simulink model "eCS_Algo_Simulation_2015b_opti - Copy"  (R2015b)
settings: Solver=ode1  StartTime=0.0  StopTime=3  FixedStep=1/80000  RelTol=1e-3
PreLoadFcn:
  | if exist('tl_preloadfcn','file'), tl_preloadfcn(gcs,402); end
PostLoadFcn:
  | , if any(exist('dsrtsu_mdlpostloadfcn', 'file') == [2, 3, 6]), try dsrtsu_mdlpostloadfcn('Execute', bdroot); catch fprintf('Error in PostLoadFcn (dsrtsu_mdlpostloadfcn) for model "%s":\n %s\n', bdroot, lasterr); end, end,
  | if exist('tl_postloadfcn','file'), tl_postloadfcn(gcs,402); end
InitFcn:
  | Omegan=1.3024e+03;
  | xi=0.9; %0.48
  | K=0.1931;
  | K1=0.0198;
  | TauLocked=0.00255;
  | TauUnLocked=0.0042;
  | Kp=1/(2*K1);
  | Ki=Kp/((TauLocked+TauUnLocked)/2);
  | if exist('tlds_init','file'), tlds_init(gcs); end
StartFcn:
  | if exist('tlds_start','file'), tlds_start(gcs); end
StopFcn:
  | if exist('tlds_stop','file'), tlds_stop(gcs); end
model workspace (MAT data in the model file):
  au8PrevExecProfile = [0 0 0 0 0 0]
values from neighbouring files (symbols this model uses):
  AccSensor = 5    [Parameter_eCS_Algo.m]
  AlgoType = 0    [Parameter_eCS_Algo.m]
  Cxy = 1*0.017    (= 0.017)    [Acc_Init_SelV1.m]
  Cxz = 1*0.017    (= 0.017)    [Acc_Init_SelV1.m]
  Cyx = 1*0.017    (= 0.017)    [Acc_Init_SelV1.m]
  Cyz = 1*0.017    (= 0.017)    [Acc_Init_SelV1.m]
  Czx = 1*0.017    (= 0.017)    [Acc_Init_SelV1.m]
  Czy = 1*0.017    (= 0.017)    [Acc_Init_SelV1.m]
  Forced_Oscillation = 0    [Parameter_eCS_Algo.m]    (also in run_Rotation_sim.m = run)
  FreqTemperature = 10    [Acc_Init_SelV1.m]
  MaxSensorOffset = 0.3    [Acc_Init_SelV1.m]
  Mean_x_noise = 4e-3    (= 0.004)    [Acc_Init_SelV1.m]
  Mean_y_noise = 4e-3    (= 0.004)    [Acc_Init_SelV1.m]
  Mean_z_noise = 4e-3    (= 0.004)    [Acc_Init_SelV1.m]
  ODR = 8000    [Acc_Init_SelV1.m]
  offsetcorrection_on_off = 0    [Parameter_eCS_Algo.m]
  phi_pulse_rotation = 0    [Parameter_eCS_Algo.m]    (also in run_Rotation_sim.m = angle)
  pulsetype = 2    [Parameter_eCS_Algo.m]    (also in run_simulation.m = j; run_simulation_ActiveX.m = j)
  Range = 4    [Acc_Init_SelV1.m]
  sensitivity_optimisation = 0    [Parameter_eCS_Algo.m]
  TempBias = 0    [Acc_Init_SelV1.m]
  TemperatureAmp = 0    [Acc_Init_SelV1.m]
  Var_x_noise = 1.84e-9    (= 1.84e-09)    [Acc_Init_SelV1.m]
  Var_y_noise = 2.025e-09    [Acc_Init_SelV1.m]
  Var_z_noise = 1.374e-09    [Acc_Init_SelV1.m]
  w_x = 2*pi*F_x    (= 376.991118431)    [Acc_Init_SelV1.m]
  w_y = 2*pi*F_y    (= 376.991118431)    [Acc_Init_SelV1.m]
  w_z = 2*pi*F_z    (= 376.991118431)    [Acc_Init_SelV1.m]
  x_max_temp_drift = 0.061    [Acc_Init_SelV1.m]
  x_offset_enable = 0    [Acc_Init_SelV1.m]
  x_run_to_run_drift = 0.0    (= 0)    [Acc_Init_SelV1.m]
  x_temp_co_drift = 0.000    (= 0)    [Acc_Init_SelV1.m]
  Xi_x = 0.7    [Acc_Init_SelV1.m]
  Xi_y = 0.7    [Acc_Init_SelV1.m]
  Xi_z = 0.7    [Acc_Init_SelV1.m]
  y_max_temp_drift = 0.061    [Acc_Init_SelV1.m]
  y_offset_enable = 0    [Acc_Init_SelV1.m]
  y_run_to_run_drift = 0.0    (= 0)    [Acc_Init_SelV1.m]
  y_temp_co_drift = 0.000    (= 0)    [Acc_Init_SelV1.m]
  z_max_temp_drift = 0.13    [Acc_Init_SelV1.m]
  z_offset_enable = 0    [Acc_Init_SelV1.m]
  z_run_to_run_drift = 0.0    (= 0)    [Acc_Init_SelV1.m]
  z_temp_co_drift = 0.000    (= 0)    [Acc_Init_SelV1.m]
undefined symbols (not defined in the file or in its folder): ddv, DiscIntNeverNeededParam, gmw_roada_x__m_s__, gmw_roada_y__m_s__, gmw_roadtime_2kHz, KSF_50_a_x, KSF_50_a_y, KSF_50_time, KSG_30_a_x, KSG_30_a_y, KSG_30_time, Meldorf_HindenburgstraAcceleration_x__m_s_2_, Meldorf_HindenburgstraAcceleration_y__m_s_2_, Meldorf_HindenburgstraAcceleration_z__m_s_2_, Meldorf_HindenburgstraTime__s_, pulse_FF27, pulse_MPDB, pulse_ODB40, pulse_ODB64, pulse_USNCAP, pulsetime_FF27, pulsetime_MPDB, pulsetime_ODB40, pulsetime_ODB64, pulsetime_USNCAP, Rauasphalt_60_a_x, Rauasphalt_60_a_y, Rauasphalt_60_time, sigbuilder_block, VW_416_2kHza_x_2kHz, VW_416_2kHza_y_2kHz, VW_416_2kHztime_2kHz
libraries: tllib x22, simulink x20, tl_autosar_lib x10, simulink_extras x7, LIB_TF_G_12_StepControl x2, LIB_TF_G_111 x1, LIB_TF_G_112 x1
(part 3 of 9)

== system eCS_Algo_Simulation_2015b_opti - Copy/FSM/Subsystem/FSM/FSM/FSM_runMainFunction ==
  drparg_b8EcsFlag : Inport  PortDimensions=1  mask(TL_Inport){data={'autosar',{'useautosarcommunication',1,'senderreceiverport','prrEcsAlgoFlag','dataelement','b8EcsFlag'},'date',738304.65103487263}}
      settings: CopyFcn=if exist('tl_reset_reviewflag') == 2, tl_reset_reviewflag(gcbh); end  DeleteFcn=if exist('delete_tlblock','file')==2,delete_tlblock(gcbh);end  NameChangeFcn=if exist('rename_tlblock','file')==2,rename_tlblock(gcbh);end  OpenFcn=if exist('tl_open_blockdlg','file')==2,tl_open_blockdlg(gcbh);else,open_system(gcbh,'parameter');end
      mask Help: eval(['if exist(''tl_online_help'',''file'') == 2, tl_online_help(''Topic'',''TL_Inport''),else, web([''jar:file:///'',matlabroot,''/help/toolbox/simulink/help.jar!/slref/' lower(get_param(gcbh,'Blocktype')) '.html''], ''-helpbrowser''),end'])
      mask Display: plot([0.2 0.35 NaN 0.65 0.8],[0 1 NaN 0 1]);
  bModeStatus : Inport  Port=2  PortDimensions=1  mask(TL_Inport){data={'autosar',{'useautosarcommunication',1,'kind',3,'interrunnablevariable','FSM_b8_ModeStatusResult','serverport','pseModeManagement'},'date',738785.60019108793}}
      settings: CopyFcn=if exist('tl_reset_reviewflag','file')==2,tl_reset_reviewflag(gcbh);end  DeleteFcn=if exist('delete_tlblock','file')==2,delete_tlblock(gcbh);end  NameChangeFcn=if exist('rename_tlblock','file')==2,rename_tlblock(gcbh);end  OpenFcn=if exist('tl_open_blockdlg','file')==2,tl_open_blockdlg(gcbh);else,open_system(gcbh,'parameter');end
      mask Help: eval(['if exist(''tl_online_help'',''file'') == 2, tl_online_help(''Topic'',''TL_Inport''),else, web([''jar:file:///'',matlabroot,''/help/toolbox/simulink/help.jar!/slref/' lower(get_param(gcbh,'Blocktype')) '.html''], ''-helpbrowser''),end'])
      mask Display: plot([0.2 0.35 NaN 0.65 0.8],[0 1 NaN 0 1]);
  ab8IsSolenoidUsed : Inport  Port=3  PortDimensions=6  mask(TL_Inport){data={'autosar',{'useautosarcommunication',1,'kind',3,'interrunnablevariable','ab8IsSolenoidUsed'},'date',738307.71878736117}}
      settings: CopyFcn=if exist('tl_reset_reviewflag') == 2, tl_reset_reviewflag(gcbh); end  DeleteFcn=if exist('delete_tlblock','file')==2,delete_tlblock(gcbh);end  NameChangeFcn=if exist('rename_tlblock','file')==2,rename_tlblock(gcbh);end  OpenFcn=if exist('tl_open_blockdlg','file')==2,tl_open_blockdlg(gcbh);else,open_system(gcbh,'parameter');end
      mask Help: eval(['if exist(''tl_online_help'',''file'') == 2, tl_online_help(''Topic'',''TL_Inport''),else, web([''jar:file:///'',matlabroot,''/help/toolbox/simulink/help.jar!/slref/' lower(get_param(gcbh,'Blocktype')) '.html''], ''-helpbrowser''),end'])
      mask Display: plot([0.2 0.35 NaN 0.65 0.8],[0 1 NaN 0 1]);
  Constant2 : Constant  Commented=on  Value=2  mask(TL_Constant){data={'date',738673.71713201387}}
      settings: CopyFcn=if exist('tl_reset_reviewflag') == 2, tl_reset_reviewflag(gcbh); end  DeleteFcn=if exist('delete_tlblock','file')==2,delete_tlblock(gcbh);end  NameChangeFcn=if exist('rename_tlblock','file')==2,rename_tlblock(gcbh);end  OpenFcn=if exist('tl_open_blockdlg','file')==2,tl_open_blockdlg(gcbh);else,open_system(gcbh,'parameter');end
      mask Help: eval(['if exist(''tl_online_help'',''file'') == 2, tl_online_help(''Topic'',''TL_Constant''),else, web([''jar:file:///'',matlabroot,''/help/toolbox/simulink/help.jar!/slref/' lower(get_param(gcbh,'Blocktype')) '.html''], ''-helpbrowser''),end'])
      mask Display: plot([-0.1, 1.05, NaN, -0.1, 1.05],[.01, .01, NaN, .99, .99]);
  Constant3 : Constant  Commented=on  Value=10  mask(TL_Constant){data={'date',738673.718190243}}
      settings: CopyFcn=if exist('tl_reset_reviewflag') == 2, tl_reset_reviewflag(gcbh); end  DeleteFcn=if exist('delete_tlblock','file')==2,delete_tlblock(gcbh);end  NameChangeFcn=if exist('rename_tlblock','file')==2,rename_tlblock(gcbh);end  OpenFcn=if exist('tl_open_blockdlg','file')==2,tl_open_blockdlg(gcbh);else,open_system(gcbh,'parameter');end
      mask Help: eval(['if exist(''tl_online_help'',''file'') == 2, tl_online_help(''Topic'',''TL_Constant''),else, web([''jar:file:///'',matlabroot,''/help/toolbox/simulink/help.jar!/slref/' lower(get_param(gcbh,'Blocktype')) '.html''], ''-helpbrowser''),end'])
      mask Display: plot([-0.1, 1.05, NaN, -0.1, 1.05],[.01, .01, NaN, .99, .99]);
  Determine Transition : Subsystem  TreatAsAtomicUnit=on
  ExecuteState : Subsystem  TreatAsAtomicUnit=on
  Logical Operator : Logic  Commented=on  Operator=OR  AllPortsSameDT=off  OutDataTypeStr=boolean  mask(TL_LogicalOperator){data={'date',738673.70713811344}}
      settings: DeleteFcn=if exist('delete_tlblock','file')==2,delete_tlblock(gcbh);end  NameChangeFcn=if exist('rename_tlblock','file')==2,rename_tlblock(gcbh);end  OpenFcn=if exist('tl_open_blockdlg','file')==2,tl_open_blockdlg(gcbh);else,open_system(gcbh,'parameter');end
      mask Help: eval(['if exist(''tl_online_help'',''file'') == 2, tl_online_help(''Topic'',''TL_LogicalOperator''),else, web([''jar:file:///'',matlabroot,''/help/toolbox/simulink/help.jar!/slref/' lower(get_param(gcbh,'Blocktype')) '.html''], ''-helpbrowser''),end'])
      mask Display: plot([-0.1, 1.05, NaN, -0.1, 1.05],[.01, .01, NaN, .99, .99]);
  Relational Operator : RelationalOperator  Commented=on  Operator===  OutDataTypeStr=boolean  mask(TL_RelationalOperator){data={'date',738673.58053900464}}
      settings: DeleteFcn=if exist('delete_tlblock','file')==2,delete_tlblock(gcbh);end  NameChangeFcn=if exist('rename_tlblock','file')==2,rename_tlblock(gcbh);end  OpenFcn=if exist('tl_open_blockdlg','file')==2,tl_open_blockdlg(gcbh);else,open_system(gcbh,'parameter');end
      mask Help: eval(['if exist(''tl_online_help'',''file'') == 2, tl_online_help(''Topic'',''TL_RelationalOperator''),else, web([''jar:file:///'',matlabroot,''/help/toolbox/simulink/help.jar!/slref/' lower(get_param(gcbh,'Blocktype')) '.html''], ''-helpbrowser''),end'])
      mask Display: plot([-0.1, 1.05, NaN, -0.1, 1.05],[.01, .01, NaN, .99, .99]);
  Relational Operator1 : RelationalOperator  Commented=on  Operator===  OutDataTypeStr=boolean  mask(TL_RelationalOperator){data={'date',738673.58053900464}}
      settings: DeleteFcn=if exist('delete_tlblock','file')==2,delete_tlblock(gcbh);end  NameChangeFcn=if exist('rename_tlblock','file')==2,rename_tlblock(gcbh);end  OpenFcn=if exist('tl_open_blockdlg','file')==2,tl_open_blockdlg(gcbh);else,open_system(gcbh,'parameter');end
      mask Help: eval(['if exist(''tl_online_help'',''file'') == 2, tl_online_help(''Topic'',''TL_RelationalOperator''),else, web([''jar:file:///'',matlabroot,''/help/toolbox/simulink/help.jar!/slref/' lower(get_param(gcbh,'Blocktype')) '.html''], ''-helpbrowser''),end'])
      mask Display: plot([-0.1, 1.05, NaN, -0.1, 1.05],[.01, .01, NaN, .99, .99]);
  Runnable : tllib/Function  data={'autosar',{'useautosarspecification',1,'softwarecomponent','AUTOLIV/SoftwareComponents/FSM/FSM','runnable','FSM_runMainFunction'},'date',738304.65103259264}  displayString=RUNNABLE
  Src2 : Subsystem  Commented=on
  old state : UnitDelay  InitialCondition=ddv('FSM/astFsm/Components/au8FsmStatesOld')  SampleTime=-1  mask(TL_UnitDelay){data={'output',{'name','$D','inheritscaling',1},'state',{'variable','FSM/astFsm/Components/au8FsmStatesOld'},'date',738331.66886591434}}
      settings: CopyFcn=if exist('tl_reset_reviewflag') == 2, tl_reset_reviewflag(gcbh); end  DeleteFcn=if exist('delete_tlblock','file')==2,delete_tlblock(gcbh);end  NameChangeFcn=if exist('rename_tlblock','file')==2,rename_tlblock(gcbh);end  OpenFcn=if exist('tl_open_blockdlg','file')==2,tl_open_blockdlg(gcbh);else,open_system(gcbh,'parameter');end
      mask Help: eval(['if exist(''tl_online_help'',''file'') == 2, tl_online_help(''Topic'',''TL_UnitDelay''),else, web([''jar:file:///'',matlabroot,''/help/toolbox/simulink/help.jar!/slref/' lower(get_param(gcbh,'Blocktype')) '.html''], ''-helpbrowser''),end'])
      mask Display: plot([-0.1, 1.05, NaN, -0.1, 1.05],[.01, .01, NaN, .99, .99]);
  scp_KL30_OV_GetTestResult : Subsystem  Commented=on  TreatAsAtomicUnit=on
  scp_KL30_UV_GetTestResult : Subsystem  Commented=on  TreatAsAtomicUnit=on
  au8FsmState : Outport  PortDimensions=6  mask(TL_Outport){data={'logdata',{'loggingmode',1},'autosar',{'useautosarcommunication',1,'senderreceiverport','psrSolenoidState','dataelement','au8SolenoidState'},'date',738314.63122943288}}
      settings: CopyFcn=if exist('tl_reset_reviewflag') == 2, tl_reset_reviewflag(gcbh); end  DeleteFcn=if exist('delete_tlblock','file')==2,delete_tlblock(gcbh);end  NameChangeFcn=if exist('rename_tlblock','file')==2,rename_tlblock(gcbh);end  OpenFcn=if exist('tl_open_blockdlg','file')==2,tl_open_blockdlg(gcbh);else,open_system(gcbh,'parameter');end
      mask Help: eval(['if exist(''tl_online_help'',''file'') == 2, tl_online_help(''Topic'',''TL_Outport''),else, web([''jar:file:///'',matlabroot,''/help/toolbox/simulink/help.jar!/slref/' lower(get_param(gcbh,'Blocktype')) '.html''], ''-helpbrowser''),end'])
      mask Display: plot([0.2 0.35 NaN 0.65 0.8],[0 1 NaN 0 1]);
  au8SelectedProfile : Outport  Port=2  PortDimensions=6  mask(TL_Outport){data={'logdata',{'loggingmode',1},'autosar',{'useautosarcommunication',1,'senderreceiverport','psrSolenoidProfile','dataelement','au8SelectedProfile'},'date',738785.47525618051}}
      settings: CopyFcn=if exist('tl_reset_reviewflag') == 2, tl_reset_reviewflag(gcbh); end  DeleteFcn=if exist('delete_tlblock','file')==2,delete_tlblock(gcbh);end  NameChangeFcn=if exist('rename_tlblock','file')==2,rename_tlblock(gcbh);end  OpenFcn=if exist('tl_open_blockdlg','file')==2,tl_open_blockdlg(gcbh);else,open_system(gcbh,'parameter');end
      mask Help: eval(['if exist(''tl_online_help'',''file'') == 2, tl_online_help(''Topic'',''TL_Outport''),else, web([''jar:file:///'',matlabroot,''/help/toolbox/simulink/help.jar!/slref/' lower(get_param(gcbh,'Blocktype')) '.html''], ''-helpbrowser''),end'])
      mask Display: plot([0.2 0.35 NaN 0.65 0.8],[0 1 NaN 0 1]);
  wires:
  drparg_b8EcsFlag/1 -> Determine Transition/1(b8EcsFlag)
  ab8IsSolenoidUsed/1 -> Determine Transition/2(ab8IsSolenoidUsed)
  Determine Transition/1(au8State) -> old state/1, ExecuteState/1(au8States), au8FsmState/1
  ExecuteState/1(au8FsmProfiles) -> au8SelectedProfile/1
  old state/1 -> Determine Transition/3(au8OldState)
  Src2/1(u8AutoTestId) -> scp_KL30_OV_GetTestResult/1(u8AutoTestId)
  scp_KL30_OV_GetTestResult/1(u8TestResult) -> Relational Operator/1
  Constant2/1 -> Relational Operator1/1, Relational Operator/2
  scp_KL30_UV_GetTestResult/1(u8TestResult) -> Relational Operator1/2
  Constant3/1 -> scp_KL30_UV_GetTestResult/1(u8AutoTestId)
  Relational Operator/1 -> Logical Operator/1
  Relational Operator1/1 -> Logical Operator/2
  bModeStatus/1 -> Determine Transition/4(bModeStatus)

== system eCS_Algo_Simulation_2015b_opti - Copy/SAD/Subsystem/SAD/SAD/SAD_Init ==
  BusCreator : BusCreator  Inputs=2
  BusCreator1 : BusCreator  Inputs=2
  Constant : Constant  Value=ddv('DIOIF/Macros/IO_Level/DIOIF_STD_HIGH')  mask(TL_Constant){data={'output',{'variable','DIOIF/Macros/IO_Level/DIOIF_STD_HIGH'},'date',738597.36695635412}}
      settings: CopyFcn=if exist('tl_reset_reviewflag') == 2, tl_reset_reviewflag(gcbh); end  DeleteFcn=if exist('delete_tlblock','file')==2,delete_tlblock(gcbh);end  NameChangeFcn=if exist('rename_tlblock','file')==2,rename_tlblock(gcbh);end  OpenFcn=if exist('tl_open_blockdlg','file')==2,tl_open_blockdlg(gcbh);else,open_system(gcbh,'parameter');end
      mask Help: eval(['if exist(''tl_online_help'',''file'') == 2, tl_online_help(''Topic'',''TL_Constant''),else, web([''jar:file:///'',matlabroot,''/help/toolbox/simulink/help.jar!/slref/' lower(get_param(gcbh,'Blocktype')) '.html''], ''-helpbrowser''),end'])
      mask Display: plot([-0.1, 1.05, NaN, -0.1, 1.05],[.01, .01, NaN, .99, .99]);
  Constant1 : Constant  Value=ddv('DIOIF/Macros/Channels/DIOIF_CH_EN_BOOST')  mask(TL_Constant){data={'output',{'variable','DIOIF/Macros/Channels/DIOIF_CH_EN_BOOST'},'date',738597.36719569447}}
      settings: CopyFcn=if exist('tl_reset_reviewflag') == 2, tl_reset_reviewflag(gcbh); end  DeleteFcn=if exist('delete_tlblock','file')==2,delete_tlblock(gcbh);end  NameChangeFcn=if exist('rename_tlblock','file')==2,rename_tlblock(gcbh);end  OpenFcn=if exist('tl_open_blockdlg','file')==2,tl_open_blockdlg(gcbh);else,open_system(gcbh,'parameter');end
      mask Help: eval(['if exist(''tl_online_help'',''file'') == 2, tl_online_help(''Topic'',''TL_Constant''),else, web([''jar:file:///'',matlabroot,''/help/toolbox/simulink/help.jar!/slref/' lower(get_param(gcbh,'Blocktype')) '.html''], ''-helpbrowser''),end'])
      mask Display: plot([-0.1, 1.05, NaN, -0.1, 1.05],[.01, .01, NaN, .99, .99]);
  Constant2 : Constant  Value=ddv('DIOIF/Macros/IO_Level/DIOIF_STD_HIGH')  mask(TL_Constant){data={'output',{'variable','DIOIF/Macros/IO_Level/DIOIF_STD_HIGH'},'date',738597.36695635412}}
      settings: CopyFcn=if exist('tl_reset_reviewflag') == 2, tl_reset_reviewflag(gcbh); end  DeleteFcn=if exist('delete_tlblock','file')==2,delete_tlblock(gcbh);end  NameChangeFcn=if exist('rename_tlblock','file')==2,rename_tlblock(gcbh);end  OpenFcn=if exist('tl_open_blockdlg','file')==2,tl_open_blockdlg(gcbh);else,open_system(gcbh,'parameter');end
      mask Help: eval(['if exist(''tl_online_help'',''file'') == 2, tl_online_help(''Topic'',''TL_Constant''),else, web([''jar:file:///'',matlabroot,''/help/toolbox/simulink/help.jar!/slref/' lower(get_param(gcbh,'Blocktype')) '.html''], ''-helpbrowser''),end'])
      mask Display: plot([-0.1, 1.05, NaN, -0.1, 1.05],[.01, .01, NaN, .99, .99]);
  Constant3 : Constant  Value=ddv('DIOIF/Macros/Channels/DIOIF_CH_EN_BOOST_2')  mask(TL_Constant){data={'output',{'variable','DIOIF/Macros/Channels/DIOIF_CH_EN_BOOST_2'},'date',738597.36739057873}}
      settings: CopyFcn=if exist('tl_reset_reviewflag') == 2, tl_reset_reviewflag(gcbh); end  DeleteFcn=if exist('delete_tlblock','file')==2,delete_tlblock(gcbh);end  NameChangeFcn=if exist('rename_tlblock','file')==2,rename_tlblock(gcbh);end  OpenFcn=if exist('tl_open_blockdlg','file')==2,tl_open_blockdlg(gcbh);else,open_system(gcbh,'parameter');end
      mask Help: eval(['if exist(''tl_online_help'',''file'') == 2, tl_online_help(''Topic'',''TL_Constant''),else, web([''jar:file:///'',matlabroot,''/help/toolbox/simulink/help.jar!/slref/' lower(get_param(gcbh,'Blocktype')) '.html''], ''-helpbrowser''),end'])
      mask Display: plot([-0.1, 1.05, NaN, -0.1, 1.05],[.01, .01, NaN, .99, .99]);
  Runnable : tllib/Function  data={'autosar',{'useautosarspecification',1,'softwarecomponent','AUTOLIV/SoftwareComponents/SAD/SAD','runnable','SAD_Init'},'date',738422.45749591431}  displayString=RUNNABLE
  EN_Boost_1 : Outport  mask(TL_BusOutport){data={'#autoscaling',2,'#message',2,'#output',2,'#logdata',2,'signals',{{'WriteChannel',{'u8ChannelID';'u8Level'}}},'autosar',{'useautosarcommunication',1,'kind',4,'clientserverport','pclDioIfServices','operation','WriteChannel'},'date',738430.41690740746}}
      settings: CopyFcn=if exist('tl_reset_reviewflag') == 2, tl_reset_reviewflag(gcbh); end  DeleteFcn=if exist('delete_tlblock','file')==2,delete_tlblock(gcbh);end  NameChangeFcn=if exist('rename_tlblock','file')==2,rename_tlblock(gcbh);end  OpenFcn=if exist('tl_open_blockdlg','file')==2,tl_open_blockdlg(gcbh);else,open_system(gcbh,'parameter');end
      mask Help: eval(['if exist(''tl_online_help'',''file'') == 2, tl_online_help(''Topic'',''TL_Outport''),else, web([''jar:file:///'',matlabroot,''/help/toolbox/simulink/help.jar!/slref/' lower(get_param(gcbh,'Blocktype')) '.html''], ''-helpbrowser''),end'])
      mask Display: plot([0.2 0.35 NaN 0.65 0.8],[0 1 NaN 0 1]);
  EN_Boost_2 : Outport  Port=2  mask(TL_BusOutport){data={'#autoscaling',2,'#message',2,'#output',2,'#logdata',2,'signals',{{'WriteChannel',{'u8ChannelID';'u8Level'}}},'autosar',{'useautosarcommunication',1,'kind',4,'clientserverport','pclDioIfServices','operation','WriteChannel'},'date',738430.41690740746}}
      settings: CopyFcn=if exist('tl_reset_reviewflag') == 2, tl_reset_reviewflag(gcbh); end  DeleteFcn=if exist('delete_tlblock','file')==2,delete_tlblock(gcbh);end  NameChangeFcn=if exist('rename_tlblock','file')==2,rename_tlblock(gcbh);end  OpenFcn=if exist('tl_open_blockdlg','file')==2,tl_open_blockdlg(gcbh);else,open_system(gcbh,'parameter');end
      mask Help: eval(['if exist(''tl_online_help'',''file'') == 2, tl_online_help(''Topic'',''TL_Outport''),else, web([''jar:file:///'',matlabroot,''/help/toolbox/simulink/help.jar!/slref/' lower(get_param(gcbh,'Blocktype')) '.html''], ''-helpbrowser''),end'])
      mask Display: plot([0.2 0.35 NaN 0.65 0.8],[0 1 NaN 0 1]);
  wires:
  Constant1/1 -> BusCreator/1  "u8ChannelID"
  Constant/1 -> BusCreator/2  "u8Level"
  BusCreator/1 -> EN_Boost_1/1  "WriteChannel"
  Constant3/1 -> BusCreator1/1  "u8ChannelID"
  Constant2/1 -> BusCreator1/2  "u8Level"
  BusCreator1/1 -> EN_Boost_2/1  "WriteChannel"

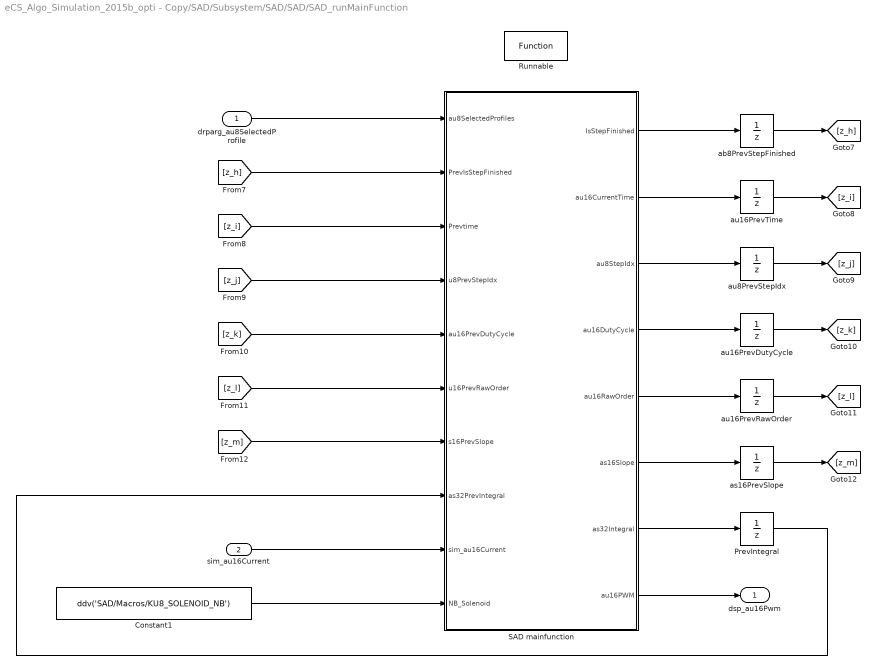
== system eCS_Algo_Simulation_2015b_opti - Copy/SAD/Subsystem/SAD/SAD/SAD_runMainFunction ==
  drparg_au8SelectedProfile : Inport  PortDimensions=6  mask(TL_Inport){data={'logdata',{'loggingmode',1},'autosar',{'useautosarcommunication',1,'senderreceiverport','prrFsmProfile','dataelement','au8SelectedProfile'},'date',738567.35573128471}}
      settings: CopyFcn=if exist('tl_reset_reviewflag') == 2, tl_reset_reviewflag(gcbh); end  DeleteFcn=if exist('delete_tlblock','file')==2,delete_tlblock(gcbh);end  NameChangeFcn=if exist('rename_tlblock','file')==2,rename_tlblock(gcbh);end  OpenFcn=if exist('tl_open_blockdlg','file')==2,tl_open_blockdlg(gcbh);else,open_system(gcbh,'parameter');end
      mask Help: eval(['if exist(''tl_online_help'',''file'') == 2, tl_online_help(''Topic'',''TL_Inport''),else, web([''jar:file:///'',matlabroot,''/help/toolbox/simulink/help.jar!/slref/' lower(get_param(gcbh,'Blocktype')) '.html''], ''-helpbrowser''),end'])
      mask Display: plot([0.2 0.35 NaN 0.65 0.8],[0 1 NaN 0 1]);
  sim_au16Current : Inport  Port=2
  Constant1 : Constant  Value=ddv('SAD/Macros/KU8_SOLENOID_NB')  mask(TL_Constant){data={'output',{'variable','SAD/Macros/KU8_SOLENOID_NB'},'date',738430.41690414352}}
      settings: CopyFcn=if exist('tl_reset_reviewflag') == 2, tl_reset_reviewflag(gcbh); end  DeleteFcn=if exist('delete_tlblock','file')==2,delete_tlblock(gcbh);end  NameChangeFcn=if exist('rename_tlblock','file')==2,rename_tlblock(gcbh);end  OpenFcn=if exist('tl_open_blockdlg','file')==2,tl_open_blockdlg(gcbh);else,open_system(gcbh,'parameter');end
      mask Help: eval(['if exist(''tl_online_help'',''file'') == 2, tl_online_help(''Topic'',''TL_Constant''),else, web([''jar:file:///'',matlabroot,''/help/toolbox/simulink/help.jar!/slref/' lower(get_param(gcbh,'Blocktype')) '.html''], ''-helpbrowser''),end'])
      mask Display: plot([-0.1, 1.05, NaN, -0.1, 1.05],[.01, .01, NaN, .99, .99]);
  PrevIntegral : UnitDelay  InitialCondition=ddv('SAD/Vars/Steps/as32PrevIntegral')  SampleTime=-1  mask(TL_UnitDelay){data={'output',{'description',['Resolution:  2^-15'],'name','$D','type','Int32','scaling','scPID'},'state',{'variable','SAD/Vars/Steps/as32PrevIntegral'},'date',738672.58140456013}}
      settings: CopyFcn=if exist('tl_reset_reviewflag') == 2, tl_reset_reviewflag(gcbh); end  DeleteFcn=if exist('delete_tlblock','file')==2,delete_tlblock(gcbh);end  NameChangeFcn=if exist('rename_tlblock','file')==2,rename_tlblock(gcbh);end  OpenFcn=if exist('tl_open_blockdlg','file')==2,tl_open_blockdlg(gcbh);else,open_system(gcbh,'parameter');end
      mask Help: eval(['if exist(''tl_online_help'',''file'') == 2, tl_online_help(''Topic'',''TL_UnitDelay''),else, web([''jar:file:///'',matlabroot,''/help/toolbox/simulink/help.jar!/slref/' lower(get_param(gcbh,'Blocktype')) '.html''], ''-helpbrowser''),end'])
      mask Display: plot([-0.1, 1.05, NaN, -0.1, 1.05],[.01, .01, NaN, .99, .99]);
  Runnable : tllib/Function  data={'autosar',{'useautosarspecification',1,'softwarecomponent','AUTOLIV/SoftwareComponents/SAD/SAD','runnable','SAD_runMainFunction'},'date',738433.36681372684}  displayString=RUNNABLE
  SAD mainfunction : Subsystem  TreatAsAtomicUnit=on
  ab8PrevStepFinished : UnitDelay  InitialCondition=ddv('SAD/Vars/Steps/b8PrevIsStepFinished')  SampleTime=-1  mask(TL_UnitDelay){data={'logdata',{'loggingmode',1},'output',{'type','Bool'},'state',{'variable','SAD/Vars/Steps/b8PrevIsStepFinished'},'date',738654.60018910875}}
      settings: CopyFcn=if exist('tl_reset_reviewflag') == 2, tl_reset_reviewflag(gcbh); end  DeleteFcn=if exist('delete_tlblock','file')==2,delete_tlblock(gcbh);end  NameChangeFcn=if exist('rename_tlblock','file')==2,rename_tlblock(gcbh);end  OpenFcn=if exist('tl_open_blockdlg','file')==2,tl_open_blockdlg(gcbh);else,open_system(gcbh,'parameter');end
      mask Help: eval(['if exist(''tl_online_help'',''file'') == 2, tl_online_help(''Topic'',''TL_UnitDelay''),else, web([''jar:file:///'',matlabroot,''/help/toolbox/simulink/help.jar!/slref/' lower(get_param(gcbh,'Blocktype')) '.html''], ''-helpbrowser''),end'])
      mask Display: plot([-0.1, 1.05, NaN, -0.1, 1.05],[.01, .01, NaN, .99, .99]);
  as16PrevSlope : UnitDelay  InitialCondition=ddv('SAD/Vars/Steps/s16PrevSlope')  SampleTime=-1  mask(TL_UnitDelay){data={'output',{'inheritscaling',1},'state',{'variable','SAD/Vars/Steps/s16PrevSlope'},'date',738654.60309630784}}
      settings: CopyFcn=if exist('tl_reset_reviewflag') == 2, tl_reset_reviewflag(gcbh); end  DeleteFcn=if exist('delete_tlblock','file')==2,delete_tlblock(gcbh);end  NameChangeFcn=if exist('rename_tlblock','file')==2,rename_tlblock(gcbh);end  OpenFcn=if exist('tl_open_blockdlg','file')==2,tl_open_blockdlg(gcbh);else,open_system(gcbh,'parameter');end
      mask Help: eval(['if exist(''tl_online_help'',''file'') == 2, tl_online_help(''Topic'',''TL_UnitDelay''),else, web([''jar:file:///'',matlabroot,''/help/toolbox/simulink/help.jar!/slref/' lower(get_param(gcbh,'Blocktype')) '.html''], ''-helpbrowser''),end'])
      mask Display: plot([-0.1, 1.05, NaN, -0.1, 1.05],[.01, .01, NaN, .99, .99]);
  au16PrevDutyCycle : UnitDelay  InitialCondition=ddv('SAD/Vars/Steps/au16PrevDutyCycle')  SampleTime=-1  mask(TL_UnitDelay){data={'output',{'type','UInt16'},'state',{'variable','SAD/Vars/Steps/au16PrevDutyCycle'},'date',738657.44661982637}}
      settings: CopyFcn=if exist('tl_reset_reviewflag') == 2, tl_reset_reviewflag(gcbh); end  DeleteFcn=if exist('delete_tlblock','file')==2,delete_tlblock(gcbh);end  NameChangeFcn=if exist('rename_tlblock','file')==2,rename_tlblock(gcbh);end  OpenFcn=if exist('tl_open_blockdlg','file')==2,tl_open_blockdlg(gcbh);else,open_system(gcbh,'parameter');end
      mask Help: eval(['if exist(''tl_online_help'',''file'') == 2, tl_online_help(''Topic'',''TL_UnitDelay''),else, web([''jar:file:///'',matlabroot,''/help/toolbox/simulink/help.jar!/slref/' lower(get_param(gcbh,'Blocktype')) '.html''], ''-helpbrowser''),end'])
      mask Display: plot([-0.1, 1.05, NaN, -0.1, 1.05],[.01, .01, NaN, .99, .99]);
  au16PrevRawOrder : UnitDelay  InitialCondition=ddv('SAD/Vars/Steps/u16PrevRawOrder')  SampleTime=-1  mask(TL_UnitDelay){data={'output',{'inheritscaling',1},'state',{'variable','SAD/Vars/Steps/u16PrevRawOrder'},'date',738654.60328724538}}
      settings: CopyFcn=if exist('tl_reset_reviewflag') == 2, tl_reset_reviewflag(gcbh); end  DeleteFcn=if exist('delete_tlblock','file')==2,delete_tlblock(gcbh);end  NameChangeFcn=if exist('rename_tlblock','file')==2,rename_tlblock(gcbh);end  OpenFcn=if exist('tl_open_blockdlg','file')==2,tl_open_blockdlg(gcbh);else,open_system(gcbh,'parameter');end
      mask Help: eval(['if exist(''tl_online_help'',''file'') == 2, tl_online_help(''Topic'',''TL_UnitDelay''),else, web([''jar:file:///'',matlabroot,''/help/toolbox/simulink/help.jar!/slref/' lower(get_param(gcbh,'Blocktype')) '.html''], ''-helpbrowser''),end'])
      mask Display: plot([-0.1, 1.05, NaN, -0.1, 1.05],[.01, .01, NaN, .99, .99]);
  au16PrevTime : UnitDelay  InitialCondition=ddv('SAD/Vars/Steps/u16PrevTime')  SampleTime=-1  mask(TL_UnitDelay){data={'logdata',{'loggingmode',1},'output',{'inheritscaling',1},'state',{'variable','SAD/Vars/Steps/u16PrevTime'},'date',738654.60352159722}}
      settings: CopyFcn=if exist('tl_reset_reviewflag') == 2, tl_reset_reviewflag(gcbh); end  DeleteFcn=if exist('delete_tlblock','file')==2,delete_tlblock(gcbh);end  NameChangeFcn=if exist('rename_tlblock','file')==2,rename_tlblock(gcbh);end  OpenFcn=if exist('tl_open_blockdlg','file')==2,tl_open_blockdlg(gcbh);else,open_system(gcbh,'parameter');end
      mask Help: eval(['if exist(''tl_online_help'',''file'') == 2, tl_online_help(''Topic'',''TL_UnitDelay''),else, web([''jar:file:///'',matlabroot,''/help/toolbox/simulink/help.jar!/slref/' lower(get_param(gcbh,'Blocktype')) '.html''], ''-helpbrowser''),end'])
      mask Display: plot([-0.1, 1.05, NaN, -0.1, 1.05],[.01, .01, NaN, .99, .99]);
  au8PrevStepIdx : UnitDelay  InitialCondition=ddv('SAD/Vars/Steps/u8PrevStepIdx')  SampleTime=-1  mask(TL_UnitDelay){data={'logdata',{'loggingmode',1},'output',{'inheritscaling',1},'state',{'variable','SAD/Vars/Steps/u8PrevStepIdx'},'date',738654.60344400466}}
      settings: CopyFcn=if exist('tl_reset_reviewflag') == 2, tl_reset_reviewflag(gcbh); end  DeleteFcn=if exist('delete_tlblock','file')==2,delete_tlblock(gcbh);end  NameChangeFcn=if exist('rename_tlblock','file')==2,rename_tlblock(gcbh);end  OpenFcn=if exist('tl_open_blockdlg','file')==2,tl_open_blockdlg(gcbh);else,open_system(gcbh,'parameter');end
      mask Help: eval(['if exist(''tl_online_help'',''file'') == 2, tl_online_help(''Topic'',''TL_UnitDelay''),else, web([''jar:file:///'',matlabroot,''/help/toolbox/simulink/help.jar!/slref/' lower(get_param(gcbh,'Blocktype')) '.html''], ''-helpbrowser''),end'])
      mask Display: plot([-0.1, 1.05, NaN, -0.1, 1.05],[.01, .01, NaN, .99, .99]);
  dsp_au16Pwm : Outport  PortDimensions=6  mask(TL_Outport){data={'logdata',{'loggingmode',1},'autosar',{'useautosarcommunication',1,'senderreceiverport','pseSolenoidPWM','dataelement','au16Pwm'},'date',738496.37130460644}}
      settings: CopyFcn=if exist('tl_reset_reviewflag') == 2, tl_reset_reviewflag(gcbh); end  DeleteFcn=if exist('delete_tlblock','file')==2,delete_tlblock(gcbh);end  NameChangeFcn=if exist('rename_tlblock','file')==2,rename_tlblock(gcbh);end  OpenFcn=if exist('tl_open_blockdlg','file')==2,tl_open_blockdlg(gcbh);else,open_system(gcbh,'parameter');end
      mask Help: eval(['if exist(''tl_online_help'',''file'') == 2, tl_online_help(''Topic'',''TL_Outport''),else, web([''jar:file:///'',matlabroot,''/help/toolbox/simulink/help.jar!/slref/' lower(get_param(gcbh,'Blocktype')) '.html''], ''-helpbrowser''),end'])
      mask Display: plot([0.2 0.35 NaN 0.65 0.8],[0 1 NaN 0 1]);
  wires:
  drparg_au8SelectedProfile/1 -> SAD mainfunction/1(au8SelectedProfiles)
  SAD mainfunction/1(IsStepFinished) -> ab8PrevStepFinished/1
  ab8PrevStepFinished/1 -> [z_h]
  [z_h] -> SAD mainfunction/2(PrevIsStepFinished)
  au16PrevTime/1 -> [z_i]
  SAD mainfunction/2(au16CurrentTime) -> au16PrevTime/1
  [z_i] -> SAD mainfunction/3(Prevtime)
  SAD mainfunction/3(au8StepIdx) -> au8PrevStepIdx/1
  au8PrevStepIdx/1 -> [z_j]
  [z_j] -> SAD mainfunction/4(u8PrevStepIdx)
  [z_k] -> SAD mainfunction/5(au16PrevDutyCycle)
  SAD mainfunction/4(au16DutyCycle) -> au16PrevDutyCycle/1
  au16PrevDutyCycle/1 -> [z_k]
  SAD mainfunction/5(au16RawOrder) -> au16PrevRawOrder/1
  SAD mainfunction/6(as16Slope) -> as16PrevSlope/1
  au16PrevRawOrder/1 -> [z_l]
  as16PrevSlope/1 -> [z_m]
  [z_l] -> SAD mainfunction/6(u16PrevRawOrder)
  [z_m] -> SAD mainfunction/7(s16PrevSlope)
  Constant1/1 -> SAD mainfunction/10(NB_Solenoid)
  SAD mainfunction/7(as32Integral) -> PrevIntegral/1
  PrevIntegral/1 -> SAD mainfunction/8(as32PrevIntegral)
  sim_au16Current/1 -> SAD mainfunction/9(sim_au16Current)
  SAD mainfunction/8(au16PWM) -> dsp_au16Pwm/1

== system eCS_Algo_Simulation_2015b_opti - Copy/eCS/Subsystem/eCS/eCS/eCS_runMainFunction ==
  drparg_stAccelMtrPerSecSqd : Inport  mask(TL_BusInport){data={'#autoscaling',3,'#message',3,'#output',3,'#logdata',3,'logdata#1',{'loggingmode',1},'logdata#2',{'loggingmode',1},'logdata#3',{'loggingmode',1},'signals',{{'stAccelMtrPerSecSqd',{'s16Ax';'s16Ay';'s16Az'}}},'autosar',{'useautosarcommunication',1,'senderreceiverport','prrAccelMtrPerSecSqd','dataelement','stAccelMtrPerSecSqd'},'date',738573.7191865046}}
      settings: CopyFcn=if exist('tl_reset_reviewflag') == 2, tl_reset_reviewflag(gcbh); end  DeleteFcn=if exist('delete_tlblock','file')==2,delete_tlblock(gcbh);end  NameChangeFcn=if exist('rename_tlblock','file')==2,rename_tlblock(gcbh);end  OpenFcn=if exist('tl_open_blockdlg','file')==2,tl_open_blockdlg(gcbh);else,open_system(gcbh,'parameter');end
      mask Help: eval(['if exist(''tl_online_help'',''file'') == 2, tl_online_help(''Topic'',''TL_Inport''),else, web([''jar:file:///'',matlabroot,''/help/toolbox/simulink/help.jar!/slref/' lower(get_param(gcbh,'Blocktype')) '.html''], ''-helpbrowser''),end'])
      mask Display: plot([0.2 0.35 NaN 0.65 0.8],[0 1 NaN 0 1]);
  drparg_b8DiagReq : Inport  Port=2  PortDimensions=1  mask(TL_Inport){data={'autosar',{'useautosarcommunication',1,'senderreceiverport','prrEcsDiagRequest','dataelement','b8DiagReq'},'date',738573.71918724535}}
      settings: CopyFcn=if exist('tl_reset_reviewflag') == 2, tl_reset_reviewflag(gcbh); end  DeleteFcn=if exist('delete_tlblock','file')==2,delete_tlblock(gcbh);end  NameChangeFcn=if exist('rename_tlblock','file')==2,rename_tlblock(gcbh);end  OpenFcn=if exist('tl_open_blockdlg','file')==2,tl_open_blockdlg(gcbh);else,open_system(gcbh,'parameter');end
      mask Help: eval(['if exist(''tl_online_help'',''file'') == 2, tl_online_help(''Topic'',''TL_Inport''),else, web([''jar:file:///'',matlabroot,''/help/toolbox/simulink/help.jar!/slref/' lower(get_param(gcbh,'Blocktype')) '.html''], ''-helpbrowser''),end'])
      mask Display: plot([0.2 0.35 NaN 0.65 0.8],[0 1 NaN 0 1]);
  BallAlgo : Subsystem  TreatAsAtomicUnit=on
  Bitwise Operator : tllib/Bitwise Operator  logicop=OR  UseBitMask=off  NumInputPorts=2  BitMask=bin2dec('11011001')  BitMaskRealWorld=Stored Integer  data={'date',738573.71919834486}
  Bus Selector : BusSelector  OutputSignals=s16Ax,s16Ay,s16Az
  Constant : Constant  Value=ddv('eCS_CFG/KS16_AZ_LOCK_THRS')  mask(TL_Constant){data={'output',{'variable','eCS_CFG/KS16_AZ_LOCK_THRS'},'date',738573.71919858793}}
      settings: CopyFcn=if exist('tl_reset_reviewflag') == 2, tl_reset_reviewflag(gcbh); end  DeleteFcn=if exist('delete_tlblock','file')==2,delete_tlblock(gcbh);end  NameChangeFcn=if exist('rename_tlblock','file')==2,rename_tlblock(gcbh);end  OpenFcn=if exist('tl_open_blockdlg','file')==2,tl_open_blockdlg(gcbh);else,open_system(gcbh,'parameter');end
      mask Help: eval(['if exist(''tl_online_help'',''file'') == 2, tl_online_help(''Topic'',''TL_Constant''),else, web([''jar:file:///'',matlabroot,''/help/toolbox/simulink/help.jar!/slref/' lower(get_param(gcbh,'Blocktype')) '.html''], ''-helpbrowser''),end'])
      mask Display: plot([-0.1, 1.05, NaN, -0.1, 1.05],[.01, .01, NaN, .99, .99]);
  Constant1 : Constant  Value=170  mask(TL_Constant){data={'date',738573.71919881948}}
      settings: CopyFcn=if exist('tl_reset_reviewflag') == 2, tl_reset_reviewflag(gcbh); end  DeleteFcn=if exist('delete_tlblock','file')==2,delete_tlblock(gcbh);end  NameChangeFcn=if exist('rename_tlblock','file')==2,rename_tlblock(gcbh);end  OpenFcn=if exist('tl_open_blockdlg','file')==2,tl_open_blockdlg(gcbh);else,open_system(gcbh,'parameter');end
      mask Help: eval(['if exist(''tl_online_help'',''file'') == 2, tl_online_help(''Topic'',''TL_Constant''),else, web([''jar:file:///'',matlabroot,''/help/toolbox/simulink/help.jar!/slref/' lower(get_param(gcbh,'Blocktype')) '.html''], ''-helpbrowser''),end'])
      mask Display: plot([-0.1, 1.05, NaN, -0.1, 1.05],[.01, .01, NaN, .99, .99]);
  Constant2 : Constant  Value=0  mask(TL_Constant){data={'date',738573.7191989352}}
      settings: CopyFcn=if exist('tl_reset_reviewflag') == 2, tl_reset_reviewflag(gcbh); end  DeleteFcn=if exist('delete_tlblock','file')==2,delete_tlblock(gcbh);end  NameChangeFcn=if exist('rename_tlblock','file')==2,rename_tlblock(gcbh);end  OpenFcn=if exist('tl_open_blockdlg','file')==2,tl_open_blockdlg(gcbh);else,open_system(gcbh,'parameter');end
      mask Help: eval(['if exist(''tl_online_help'',''file'') == 2, tl_online_help(''Topic'',''TL_Constant''),else, web([''jar:file:///'',matlabroot,''/help/toolbox/simulink/help.jar!/slref/' lower(get_param(gcbh,'Blocktype')) '.html''], ''-helpbrowser''),end'])
      mask Display: plot([-0.1, 1.05, NaN, -0.1, 1.05],[.01, .01, NaN, .99, .99]);
  Constant3 : Constant  mask(TL_Constant){data={'date',738573.71919905092}}
      settings: CopyFcn=if exist('tl_reset_reviewflag') == 2, tl_reset_reviewflag(gcbh); end  DeleteFcn=if exist('delete_tlblock','file')==2,delete_tlblock(gcbh);end  NameChangeFcn=if exist('rename_tlblock','file')==2,rename_tlblock(gcbh);end  OpenFcn=if exist('tl_open_blockdlg','file')==2,tl_open_blockdlg(gcbh);else,open_system(gcbh,'parameter');end
      mask Help: eval(['if exist(''tl_online_help'',''file'') == 2, tl_online_help(''Topic'',''TL_Constant''),else, web([''jar:file:///'',matlabroot,''/help/toolbox/simulink/help.jar!/slref/' lower(get_param(gcbh,'Blocktype')) '.html''], ''-helpbrowser''),end'])
      mask Display: plot([-0.1, 1.05, NaN, -0.1, 1.05],[.01, .01, NaN, .99, .99]);
  Crash Acceleration : Subsystem  TreatAsAtomicUnit=on
  Data Type Conversion : DataTypeConversion  OutDataTypeStr=boolean
  Data Type Conversion1 : DataTypeConversion  OutDataTypeStr=boolean
  Mux : Mux  Inputs=2
  Relational Operator : RelationalOperator  OutDataTypeStr=boolean  mask(TL_RelationalOperator){data={'date',738686.73485479166}}
      settings: DeleteFcn=if exist('delete_tlblock','file')==2,delete_tlblock(gcbh);end  NameChangeFcn=if exist('rename_tlblock','file')==2,rename_tlblock(gcbh);end  OpenFcn=if exist('tl_open_blockdlg','file')==2,tl_open_blockdlg(gcbh);else,open_system(gcbh,'parameter');end
      mask Help: eval(['if exist(''tl_online_help'',''file'') == 2, tl_online_help(''Topic'',''TL_RelationalOperator''),else, web([''jar:file:///'',matlabroot,''/help/toolbox/simulink/help.jar!/slref/' lower(get_param(gcbh,'Blocktype')) '.html''], ''-helpbrowser''),end'])
      mask Display: plot([-0.1, 1.05, NaN, -0.1, 1.05],[.01, .01, NaN, .99, .99]);
  Relational Operator1 : RelationalOperator  Operator===  OutDataTypeStr=boolean  mask(TL_RelationalOperator){data={'date',738573.71920568286}}
      settings: DeleteFcn=if exist('delete_tlblock','file')==2,delete_tlblock(gcbh);end  NameChangeFcn=if exist('rename_tlblock','file')==2,rename_tlblock(gcbh);end  OpenFcn=if exist('tl_open_blockdlg','file')==2,tl_open_blockdlg(gcbh);else,open_system(gcbh,'parameter');end
      mask Help: eval(['if exist(''tl_online_help'',''file'') == 2, tl_online_help(''Topic'',''TL_RelationalOperator''),else, web([''jar:file:///'',matlabroot,''/help/toolbox/simulink/help.jar!/slref/' lower(get_param(gcbh,'Blocktype')) '.html''], ''-helpbrowser''),end'])
      mask Display: plot([-0.1, 1.05, NaN, -0.1, 1.05],[.01, .01, NaN, .99, .99]);
  Runnable : tllib/Function  data={'autosar',{'useautosarspecification',1,'softwarecomponent','AUTOLIV/SoftwareComponents/eCS/eCS','runnable','eCS_runMainFunction'},'date',738492.60443505784}  displayString=RUNNABLE
  Switch : Switch  Criteria=u2 ~= 0  mask(TL_Switch){data={'output',{'type','Bool'},'date',738573.7192059143}}
      settings: CopyFcn=if exist('tl_reset_reviewflag') == 2, tl_reset_reviewflag(gcbh); end  DeleteFcn=if exist('delete_tlblock','file')==2,delete_tlblock(gcbh);end  NameChangeFcn=if exist('rename_tlblock','file')==2,rename_tlblock(gcbh);end  OpenFcn=if exist('tl_open_blockdlg','file')==2,tl_open_blockdlg(gcbh);else,open_system(gcbh,'parameter');end
      mask Help: eval(['if exist(''tl_online_help'',''file'') == 2, tl_online_help(''Topic'',''TL_Switch''),else, web([''jar:file:///'',matlabroot,''/help/toolbox/simulink/help.jar!/slref/' lower(get_param(gcbh,'Blocktype')) '.html''], ''-helpbrowser''),end'])
      mask Display: plot([-0.1, 1.05, NaN, -0.1, 1.05],[.01, .01, NaN, .99, .99]);
  eCS Latch Output : Subsystem  TreatAsAtomicUnit=on
  mToMm : Gain  Gain=ddv('MToMM')  mask(TL_Gain){data={'output',{'type','UInt16','lsb',2^-15,'unit','m'},'gain',{'variable','MToMM'},'date',738573.71921030094}}
      settings: CopyFcn=if exist('tl_reset_reviewflag') == 2, tl_reset_reviewflag(gcbh); end  DeleteFcn=if exist('delete_tlblock','file')==2,delete_tlblock(gcbh);end  NameChangeFcn=if exist('rename_tlblock','file')==2,rename_tlblock(gcbh);end  OpenFcn=if exist('tl_open_blockdlg','file')==2,tl_open_blockdlg(gcbh);else,open_system(gcbh,'parameter');end
      mask Help: eval(['if exist(''tl_online_help'',''file'') == 2, tl_online_help(''Topic'',''TL_Gain''),else, web([''jar:file:///'',matlabroot,''/help/toolbox/simulink/help.jar!/slref/' lower(get_param(gcbh,'Blocktype')) '.html''], ''-helpbrowser''),end'])
      mask Display: plot([0, .88, 0],[.05, .5, .93]);
  mergedTrigger : Logic  Operator=OR  AllPortsSameDT=off  OutDataTypeStr=boolean  mask(TL_LogicalOperator){data={'date',738573.71921041666}}
      settings: DeleteFcn=if exist('delete_tlblock','file')==2,delete_tlblock(gcbh);end  NameChangeFcn=if exist('rename_tlblock','file')==2,rename_tlblock(gcbh);end  OpenFcn=if exist('tl_open_blockdlg','file')==2,tl_open_blockdlg(gcbh);else,open_system(gcbh,'parameter');end
      mask Help: eval(['if exist(''tl_online_help'',''file'') == 2, tl_online_help(''Topic'',''TL_LogicalOperator''),else, web([''jar:file:///'',matlabroot,''/help/toolbox/simulink/help.jar!/slref/' lower(get_param(gcbh,'Blocktype')) '.html''], ''-helpbrowser''),end'])
      mask Display: plot([-0.1, 1.05, NaN, -0.1, 1.05],[.01, .01, NaN, .99, .99]);
  dsp_b8EcsFlag : Outport  PortDimensions=1  mask(TL_Outport){data={'autosar',{'useautosarcommunication',1,'senderreceiverport','psrEcsAlgoData','dataelement','b8EcsFlag'},'date',738573.71921065974}}
      settings: CopyFcn=if exist('tl_reset_reviewflag') == 2, tl_reset_reviewflag(gcbh); end  DeleteFcn=if exist('delete_tlblock','file')==2,delete_tlblock(gcbh);end  NameChangeFcn=if exist('rename_tlblock','file')==2,rename_tlblock(gcbh);end  OpenFcn=if exist('tl_open_blockdlg','file')==2,tl_open_blockdlg(gcbh);else,open_system(gcbh,'parameter');end
      mask Help: eval(['if exist(''tl_online_help'',''file'') == 2, tl_online_help(''Topic'',''TL_Outport''),else, web([''jar:file:///'',matlabroot,''/help/toolbox/simulink/help.jar!/slref/' lower(get_param(gcbh,'Blocktype')) '.html''], ''-helpbrowser''),end'])
      mask Display: plot([0.2 0.35 NaN 0.65 0.8],[0 1 NaN 0 1]);
  dsp_u16BallPosition : Outport  Port=2  PortDimensions=1  mask(TL_Outport){data={'logdata',{'loggingmode',1},'autosar',{'useautosarcommunication',1,'senderreceiverport','psrEcsAlgoData','dataelement','u16BallPosition'},'date',738573.71921085648}}
      settings: CopyFcn=if exist('tl_reset_reviewflag') == 2, tl_reset_reviewflag(gcbh); end  DeleteFcn=if exist('delete_tlblock','file')==2,delete_tlblock(gcbh);end  NameChangeFcn=if exist('rename_tlblock','file')==2,rename_tlblock(gcbh);end  OpenFcn=if exist('tl_open_blockdlg','file')==2,tl_open_blockdlg(gcbh);else,open_system(gcbh,'parameter');end
      mask Help: eval(['if exist(''tl_online_help'',''file'') == 2, tl_online_help(''Topic'',''TL_Outport''),else, web([''jar:file:///'',matlabroot,''/help/toolbox/simulink/help.jar!/slref/' lower(get_param(gcbh,'Blocktype')) '.html''], ''-helpbrowser''),end'])
      mask Display: plot([0.2 0.35 NaN 0.65 0.8],[0 1 NaN 0 1]);
  wires:
  drparg_stAccelMtrPerSecSqd/1 -> Bus Selector/1
  drparg_b8DiagReq/1 -> Relational Operator1/2
  mToMm/1 -> dsp_u16BallPosition/1
  Mux/1 -> BallAlgo/1(Pulses(x,y))
  Bus Selector/2 -> Crash Acceleration/2(Ay), Mux/2  "<s16Ay>"
  BallAlgo/1(BallPosition(m)) -> mToMm/1
  Crash Acceleration/1(b8CrashTrigger) -> mergedTrigger/2
  BallAlgo/2(BallPosTrigger) -> mergedTrigger/1
  Bus Selector/3 -> Relational Operator/1  "<s16Az>"
  Constant/1 -> Relational Operator/2
  Relational Operator/1 -> eCS Latch Output/2(b8IsAzLockReq)
  mergedTrigger/1 -> eCS Latch Output/1(b8eCSTrigger)
  Relational Operator1/1 -> Switch/2
  Constant1/1 -> Relational Operator1/1
  Constant2/1 -> Switch/3
  eCS Latch Output/1(b8eCSTriggerFiltered) -> Data Type Conversion/1
  Bitwise Operator/1 -> dsp_b8EcsFlag/1
  Constant3/1 -> Switch/1
  Switch/1 -> Data Type Conversion1/1
  Data Type Conversion/1 -> Bitwise Operator/1
  Data Type Conversion1/1 -> Bitwise Operator/2
  Bus Selector/1 -> Crash Acceleration/1(Ax), Mux/1  "<s16Ax>"

== system eCS_Algo_Simulation_2015b_opti - Copy/FSM/Subsystem/FSM/FSM/FSM_runCheckModeStatus/Src2 ==
  Const : Constant  Value=0  mask(TL_Constant){data={'date',738776.66828796291}}
      settings: CopyFcn=if exist('tl_reset_reviewflag') == 2, tl_reset_reviewflag(gcbh); end  DeleteFcn=if exist('delete_tlblock','file')==2,delete_tlblock(gcbh);end  NameChangeFcn=if exist('rename_tlblock','file')==2,rename_tlblock(gcbh);end  OpenFcn=if exist('tl_open_blockdlg','file')==2,tl_open_blockdlg(gcbh);else,open_system(gcbh,'parameter');end
      mask Help: eval(['if exist(''tl_online_help'',''file'') == 2, tl_online_help(''Topic'',''TL_Constant''),else, web([''jar:file:///'',matlabroot,''/help/toolbox/simulink/help.jar!/slref/' lower(get_param(gcbh,'Blocktype')) '.html''], ''-helpbrowser''),end'])
      mask Display: plot([-0.1, 1.05, NaN, -0.1, 1.05],[.01, .01, NaN, .99, .99]);
  bModeStatus : Outport
  wires:
  Const/1 -> bModeStatus/1  "bModeStatus"
